simulink model "cv_3_sim"  (R2019b)
settings: Solver=FixedStepAuto  StartTime=0.0  StopTime=Tsim  FixedStep=Ts  RelTol=1e-3
values from neighbouring files (symbols this model uses):
  beta = 0.5*sqrt(g/l)    [cv_3.m]    (also in prev_char.m)
  g = 9.81    [cv_3.m]    (also in prev_char.m)
  l = 1    [cv_3.m]    (also in prev_char.m)
  m = 1    [cv_3.m]    (also in prev_char.m)
  omega_0 = 0    [cv_3.m]    (also in prev_char.m)
  phi_0 = 0.25    [cv_3.m]    (also in prev_char.m = 0)
undefined symbols (not defined in the file or in its folder): u_0
settings Model: Creator=Martin Dodek  LastModifiedBy=Martin Dodek

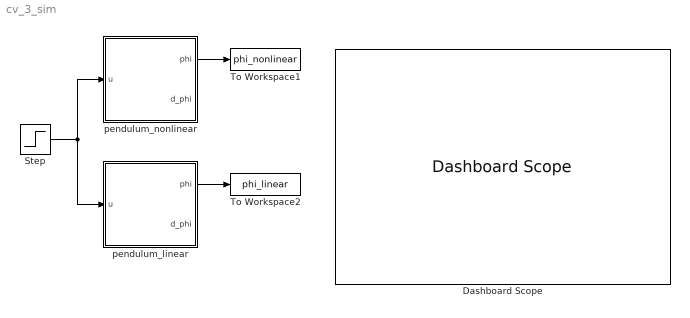
== system cv_3_sim ==
  Dashboard Scope : DashboardScope
  Step : Step  Time=5  After=5  SampleTime=0
  To Workspace1 : ToWorkspace  VariableName=phi_nonlinear  SampleTime=-1
  To Workspace2 : ToWorkspace  VariableName=phi_linear  SampleTime=-1
  pendulum_linear : Subsystem
  pendulum_nonlinear : Subsystem
  wires:
  Step/1 -> pendulum_linear/1(u), pendulum_nonlinear/1(u)
  pendulum_nonlinear/1(phi) -> To Workspace1/1
  pendulum_linear/1(phi) -> To Workspace2/1

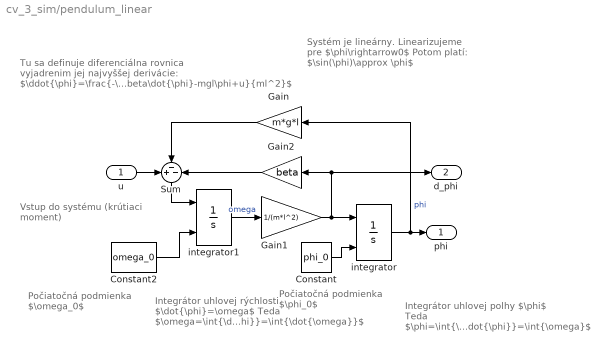
== system cv_3_sim/pendulum_linear ==
  note: Systém je lineárny. Linearizujeme pre $\phi\rightarrow0$
      | Potom platí:
      | $\sin(\phi)\approx \phi$
  note: Tu sa definuje diferenciálna rovnica vyjadrenim jej najvyššej derivácie:
      | $\ddot{\phi}=\frac{-\beta\dot{\phi}-mgl\phi+u}{ml^2}$
  note: Integrátor uhlovej polhy $\phi$
      | Teda $\phi=\int{\dot{\phi}}=\int{\omega}$
  note: Integrátor uhlovej rýchlosti $\dot{\phi}=\omega$
      | Teda $\omega=\int{\ddot{\phi}}=\int{\dot{\omega}}$
  note: Počiatočná podmienka
      | $\omega_0$
  note: Počiatočná podmienka
      | $\phi_0$
  note: Vstup do systému (krútiaci moment)
  u : Inport
  Constant : Constant  Value=phi_0
  Constant2 : Constant  Value=omega_0
  Gain : Gain  Gain=m*g*l
  Gain1 : Gain  Gain=1/(m*l^2)
  Gain2 : Gain  Gain=beta
  Sum : Sum  Inputs=+--
  integrator : Integrator  InitialConditionSource=external  InitialCondition=u_0
  integrator1 : Integrator  InitialConditionSource=external  InitialCondition=u_0
  phi : Outport
  d_phi : Outport  Port=2
  wires:
  u/1 -> Sum/1
  Gain1/1 -> d_phi/1, Gain2/1, integrator/1
  Constant2/1 -> integrator1/2
  integrator1/1 -> Gain1/1  "omega"
  Constant/1 -> integrator/2
  Gain2/1 -> Sum/3
  integrator/1 -> Gain/1, phi/1  "phi"
  Gain/1 -> Sum/2
  Sum/1 -> integrator1/1

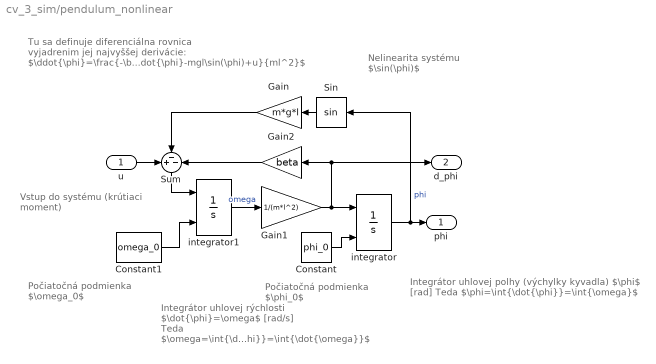
== system cv_3_sim/pendulum_nonlinear ==
  note: Počiatočná podmienka
      | $\phi_0$
  note: Počiatočná podmienka
      | $\omega_0$
  note: Integrátor uhlovej polhy (výchylky kyvadla) $\phi$ [rad]
      | Teda $\phi=\int{\dot{\phi}}=\int{\omega}$
  note: Nelinearita systému
      | $\sin(\phi)$
  note: Tu sa definuje diferenciálna rovnica vyjadrenim jej najvyššej derivácie:
      | $\ddot{\phi}=\frac{-\beta\dot{\phi}-mgl\sin(\phi)+u}{ml^2}$
  note: Vstup do systému (krútiaci moment)
  note: Integrátor uhlovej rýchlosti $\dot{\phi}=\omega$ [rad/s]
      | Teda $\omega=\int{\ddot{\phi}}=\int{\dot{\omega}}$
  u : Inport
  Constant : Constant  Value=phi_0
  Constant1 : Constant  Value=omega_0
  Gain : Gain  Gain=m*g*l
  Gain1 : Gain  Gain=1/(m*l^2)
  Gain2 : Gain  Gain=beta
  Sin : Trigonometry
  Sum : Sum  Inputs=+--
  integrator : Integrator  InitialConditionSource=external  InitialCondition=u_0
  integrator1 : Integrator  InitialConditionSource=external  InitialCondition=u_0
  phi : Outport
  d_phi : Outport  Port=2
  wires:
  integrator/1 -> Sin/1, phi/1  "phi"
  Constant1/1 -> integrator1/2
  integrator1/1 -> Gain1/1  "omega"
  Constant/1 -> integrator/2
  Sin/1 -> Gain/1
  Gain1/1 -> d_phi/1, Gain2/1, integrator/1
  Sum/1 -> integrator1/1
  u/1 -> Sum/1
  Gain2/1 -> Sum/3
  Gain/1 -> Sum/2
